simulink model "Linear_Moving_Setpoint_SS_PID"  (R2021b)
settings: Solver=VariableStepAuto  StartTime=tspan(1)  StopTime=tspan(2)  RelTol=1e-9
undefined symbols (not defined in the file): K1, K2, r_sim, x_0
settings Model: Creator=domin  LastModifiedBy=domin
settings SolverCC: AlgebraicLoopSolver=TrustRegion
settings DebuggingCC: SFMachineParentedDataDiag=warning

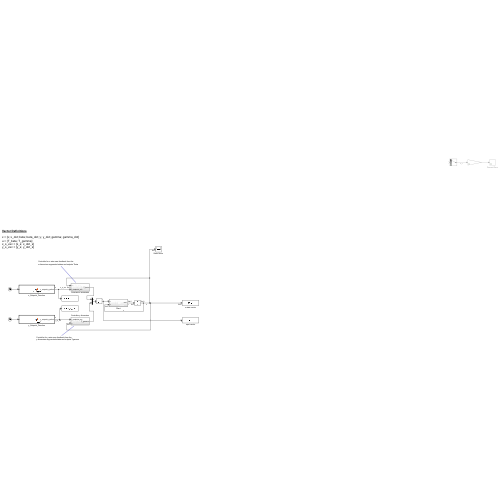
[thumbnail: Simulink's stored preview of the top-level diagram]
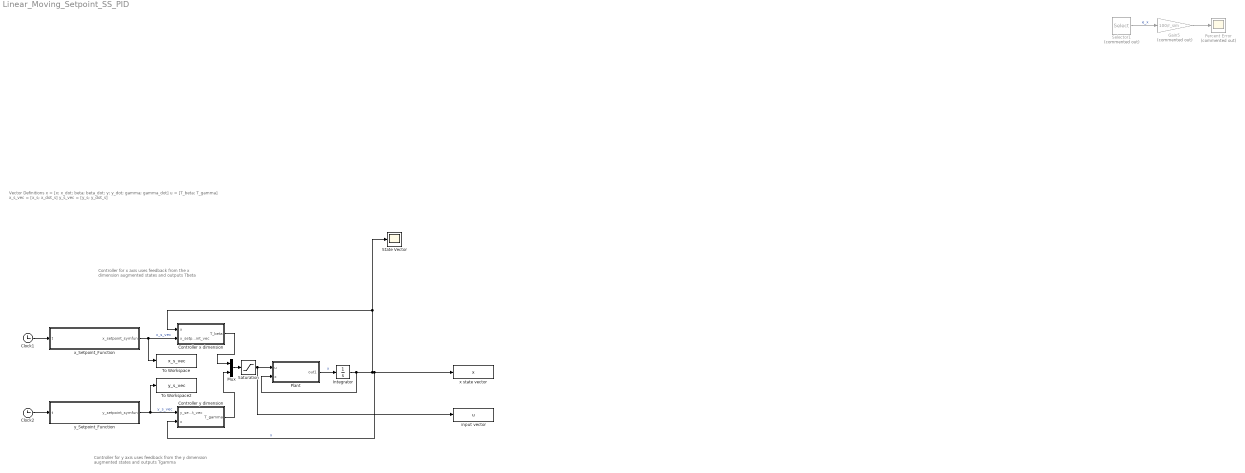
== system Linear_Moving_Setpoint_SS_PID ==
  note: Controller for y axis uses feedback from the
      | y dimension augmented states and outputs Tgamma
  note: Vector Definitions
      |
      | x = [x; x_dot; beta; beta_dot; y; y_dot; gamma; gamma_dot]
      | u = [T_beta; T_gamma]
      | x_s_vec = [x_s; x_dot_s]
      | y_s_vec = [y_s; y_dot_s]
  note: Controller for x axis uses feedback from the
      | x dimension augmented states and outputs Tbeta
  Clock1 : Clock
  Clock2 : Clock
  Controller x dimension : Subsystem
  Controller y dimension : Subsystem
  Gain5 : Gain  Commented=on  Gain=100/r_sim
  Integrator : Integrator  InitialCondition=x_0
  Mux : Mux  Inputs=2
  Percent Error : Scope  Commented=on
  Plant : Subsystem
  Saturation : Saturate  UpperLimit=73/1000  LowerLimit=-73/1000
  Selector1 : Selector  Commented=on  InputPortWidth=5  IndexOptions=Index vector (dialog)  Indices=[1]  OutputSizes=1
  State Vector : Scope
  To Workspace : ToWorkspace  VariableName=x_s_vec  SampleTime=-1
  To Workspace2 : ToWorkspace  VariableName=y_s_vec  SampleTime=-1
  input vector : ToWorkspace  VariableName=u  SampleTime=-1
  x state vector : ToWorkspace  VariableName=x  SampleTime=-1
  x_Setpoint_Function : MATLAB Function  TreatAsAtomicUnit=on
  y_Setpoint_Function : MATLAB Function  TreatAsAtomicUnit=on
  wires:
  x_Setpoint_Function/1(x_setpoint_symfun) -> To Workspace/1, Controller x dimension/2(x_setpoint_vec)  "x_s_vec"
  Integrator/1 -> Plant/2(x), Controller y dimension/2(x), x state vector/1, Controller x dimension/1(x), State Vector/1  "x"
  Plant/1(out1) -> Integrator/1  "x"
  Clock1/1 -> x_Setpoint_Function/1(t)
  Gain5/1 -> Percent Error/1
  Selector1/1 -> Gain5/1  "e_x"
  Clock2/1 -> y_Setpoint_Function/1(t)
  Mux/1 -> Saturation/1
  Controller x dimension/1(T_beta) -> Mux/1
  Controller y dimension/1(T_gamma) -> Mux/2
  y_Setpoint_Function/1(y_setpoint_symfun) -> To Workspace2/1, Controller y dimension/1(y_setpoint_vec)  "y_s_vec"
  Saturation/1 -> Plant/1(u), input vector/1

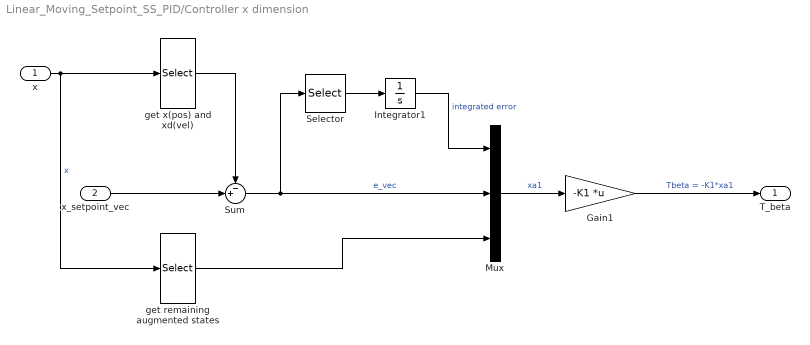
== system Linear_Moving_Setpoint_SS_PID/Controller x dimension ==
  x : Inport
  x_setpoint_vec : Inport  Port=2
  Gain1 : Gain  Gain=-K1  Multiplication=Matrix(K*u)
  Integrator1 : Integrator
  Mux : Mux  Inputs=3
  Selector : Selector  InputPortWidth=2  IndexOptions=Index vector (dialog)  Indices=[1 ]  OutputSizes=1
  Sum : Sum  Inputs=-+|
  get remaining augmented states : Selector  InputPortWidth=8  IndexOptions=Index vector (dialog)  Indices=[3,4]  OutputSizes=1
  get x(pos) and xd(vel) : Selector  InputPortWidth=8  IndexOptions=Index vector (dialog)  Indices=[1 2]  OutputSizes=1
  T_beta : Outport
  wires:
  get remaining augmented states/1 -> Mux/3
  Gain1/1 -> T_beta/1  "Tbeta = -K1*xa1"
  get x(pos) and xd(vel)/1 -> Sum/1
  Mux/1 -> Gain1/1  "xa1"
  Sum/1 -> Selector/1, Mux/2  "e_vec"
  x_setpoint_vec/1 -> Sum/2
  x/1 -> get x(pos) and xd(vel)/1, get remaining augmented states/1  "x"
  Selector/1 -> Integrator1/1
  Integrator1/1 -> Mux/1  "integrated error"

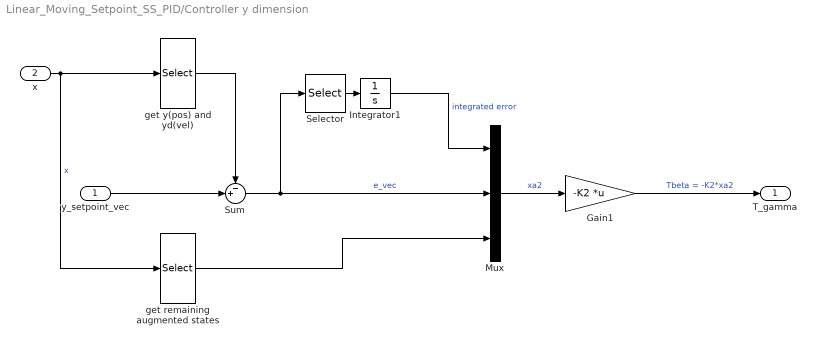
== system Linear_Moving_Setpoint_SS_PID/Controller y dimension ==
  y_setpoint_vec : Inport
  x : Inport  Port=2
  Gain1 : Gain  Gain=-K2  Multiplication=Matrix(K*u)
  Integrator1 : Integrator
  Mux : Mux  Inputs=3
  Selector : Selector  InputPortWidth=2  IndexOptions=Index vector (dialog)  Indices=[1 ]  OutputSizes=1
  Sum : Sum  Inputs=-+|
  get remaining augmented states : Selector  InputPortWidth=8  IndexOptions=Index vector (dialog)  Indices=[7,8]  OutputSizes=1
  get y(pos) and yd(vel) : Selector  InputPortWidth=8  IndexOptions=Index vector (dialog)  Indices=[5 6]  OutputSizes=1
  T_gamma : Outport
  wires:
  Integrator1/1 -> Mux/1  "integrated error"
  x/1 -> get y(pos) and yd(vel)/1, get remaining augmented states/1  "x"
  Gain1/1 -> T_gamma/1  "Tbeta = -K2*xa2"
  get y(pos) and yd(vel)/1 -> Sum/1
  Mux/1 -> Gain1/1  "xa2"
  get remaining augmented states/1 -> Mux/3
  Selector/1 -> Integrator1/1
  Sum/1 -> Selector/1, Mux/2  "e_vec"
  y_setpoint_vec/1 -> Sum/2

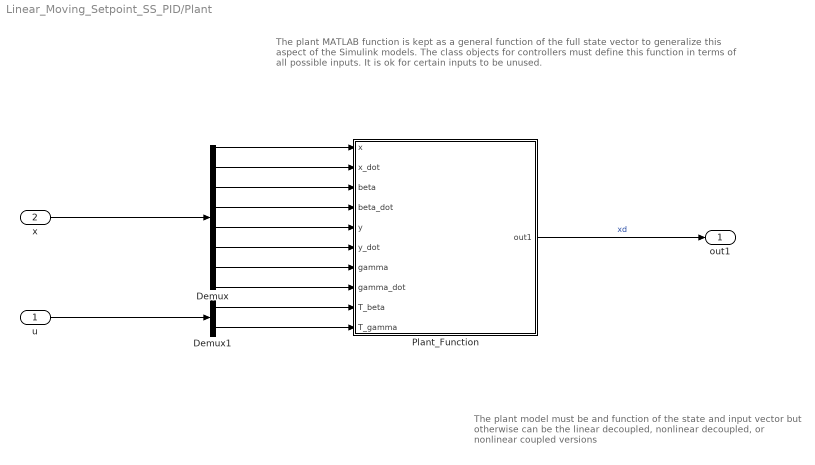
== system Linear_Moving_Setpoint_SS_PID/Plant ==
  note: The plant MATLAB function is kept as a general function of the full state vector
      | to generalize this aspect of the Simulink models. The class objects for controllers must define this function in terms of all possible inputs. It is ok for certain inputs to be unused.
  note: The plant model must be and function of the state and input vector
      |  but otherwise can be the linear decoupled, nonlinear decoupled,
      | or nonlinear coupled versions
  u : Inport
  x : Inport  Port=2
  Demux : Demux  Outputs=8
  Demux1 : Demux  Outputs=2
  Plant_Function : MATLAB Function  TreatAsAtomicUnit=on
  out1 : Outport
  wires:
  Demux1/1 -> Plant_Function/9(T_beta)
  Demux1/2 -> Plant_Function/10(T_gamma)
  Demux/5 -> Plant_Function/5(y)
  Demux/8 -> Plant_Function/8(gamma_dot)
  Demux/7 -> Plant_Function/7(gamma)
  Demux/1 -> Plant_Function/1(x)
  Demux/3 -> Plant_Function/3(beta)
  Demux/4 -> Plant_Function/4(beta_dot)
  Demux/2 -> Plant_Function/2(x_dot)
  Demux/6 -> Plant_Function/6(y_dot)
  x/1 -> Demux/1
  Plant_Function/1(out1) -> out1/1  "xd"
  u/1 -> Demux1/1

== matlab function Linear_Moving_Setpoint_SS_PID/Plant/Plant_Function ==
  data: x input; out1 output size=8; x_dot input; beta input; beta_dot input; y input; y_dot input; gamma input; gamma_dot input; T_beta input; T_gamma input
function out1 = xdot(x,x_dot,beta,beta_dot,y,y_dot,gamma,gamma_dot,T_beta,T_gamma)
%#codegen

%    This function was generated by the Symbolic Math Toolbox version 9.0.
%    08-Nov-2021 16:28:32

t2 = cos(beta);
t3 = cos(gamma);
t4 = sin(beta);
t5 = sin(gamma);
t6 = beta_dot.^2;
t7 = gamma_dot.^2;
t8 = x.^2;
t9 = x.^3;
t10 = y.^2;
t11 = y.^3;
t13 = y.^5;
t12 = t10.^2;
t14 = t3.^2;
t15 = t3.^3;
t17 = t3.^5;
t19 = t5.^2;
t20 = t5.^3;
t22 = t5.^5;
t29 = t3.*t5.*t8.*y.*6.615e-4;
t33 = t3.*t5.*y.*3.93855e-4;
t16 = t14.^2;
t18 = t14.^3;
t21 = t19.^2;
t24 = t3.*t11.*t20.*6.3e-3;
t25 = t5.*t11.*t15.*6.3e-3;
t27 = t8.*t19.*3.948e-3;
t28 = t12.*t14.*t19.*(6.3e+1./1.0e+3);
t31 = -t29;
t32 = t8.*t10.*t14.*t19.*(6.3e+1./1.0e+3);
t34 = t10.*t19.*3.93855e-3;
t35 = t8.*t14.*1.3784925e-2;
t37 = t3.*t8.*t20.*y.*6.9615e-3;
t38 = t5.*t8.*t15.*y.*6.9615e-3;
t39 = t3.*t20.*y.*1.53621e-4;
t40 = t5.*t15.*y.*1.53621e-4;
t44 = t14.*1.197923111e-3;
t45 = t8.*t14.*t19.*6.858495e-3;
t46 = t19.*6.079151925e-7;
t48 = t10.*t14.*t19.*2.070759405e-2;
t49 = t14.*t19.*4.674805062135e-4;
t23 = t12.*t21.*(6.3e+1./1.0e+3);
t26 = t8.*t10.*t21.*(6.3e+1./1.0e+3);
t30 = t8.*t21.*1.48176e-3;
t36 = t10.*t16.*1.916166e-2;
t41 = t8.*t16.*5.376735e-3;
t42 = t10.*t21.*1.54593405e-3;
t43 = t16.*4.672433922e-4;
t47 = t21.*2.371140135e-7;
t50 = t23+t24+t25+t26+t27+t28+t30+t31+t32+t33+t34+t35+t36+t37+t38+t39+t40+t41+t42+t43+t44+t45+t46+t47+t48+t49;
t51 = 1.0./t50;
et1 = T_beta.*t3.*(-2.123534875e-2)-T_beta.*t15.*8.28273225e-3+t4.*t14.*4.8049835404725e-3+t4.*t16.*1.8741576886695e-3+t4.*t19.*4.259748598875e-6+t4.*t21.*1.661491766025e-6-T_beta.*t3.*t19.*8.28273225e-3;
et2 = T_beta.*t10.*t15.*(-3.39675e-1)-T_beta.*t11.*t20.*(2.1e+1./4.0)+beta_dot.*gamma_dot.*t20.*5.4364987215e-8+beta_dot.*gamma_dot.*t22.*2.1204767493e-8-T_beta.*t5.*y.*3.282125e-1-T_beta.*t20.*y.*1.280175e-1-beta_dot.*t20.*y_dot.*1.04214033e-6-beta_dot.*t22.*y_dot.*4.06481166e-7;
et3 = t4.*t8.*t14.*9.659293875e-2+t4.*t8.*t16.*3.767555025e-2+t6.*t9.*t14.*9.846375e-3+t4.*t10.*t16.*7.685924085e-2+t4.*t8.*t19.*2.76642e-2+t6.*t9.*t16.*3.840525e-3+t4.*t8.*t21.*1.0382904e-2+t6.*t9.*t19.*2.82e-3+t4.*t10.*t21.*6.81378075e-5;
et4 = t6.*t9.*t21.*1.0584e-3+t4.*t14.*t19.*1.875819180435525e-3-t2.*t3.*x.*6.249563137125e-3-t2.*t15.*x.*2.437608101175e-3+t6.*t14.*x.*8.4655850125e-4+t7.*t14.*x.*3.854215798125e-5;
et5 = t6.*t16.*x.*3.6873769573125e-4+t7.*t16.*x.*1.503315903375e-5+t6.*t18.*x.*1.503315903375e-5+t6.*t19.*x.*4.342251375e-7+t6.*t21.*x.*1.693671525e-7-T_beta.*t5.*t11.*t14.*(2.1e+1./4.0)-T_beta.*t3.*t10.*t19.*3.39675e-1;
et6 = beta_dot.*gamma_dot.*t5.*t14.*(-3.66123403597875e-6)-beta_dot.*gamma_dot.*t5.*t16.*1.42804441695825e-6+beta_dot.*gamma_dot.*t8.*t20.*3.53064e-4-beta_dot.*gamma_dot.*t11.*t17.*2.708265e-2+beta_dot.*gamma_dot.*t8.*t22.*1.3251168e-4+beta_dot.*gamma_dot.*t10.*t20.*4.1354775e-5+beta_dot.*gamma_dot.*t10.*t22.*1.69998129e-5;
et7 = beta_dot.*gamma_dot.*t12.*t22.*6.615e-4-beta_dot.*gamma_dot.*t14.*t20.*1.40683964946525e-6+T_gamma.*t3.*t5.*x.*4.8525e-3-T_beta.*t5.*t14.*y.*1.280175e-1-beta_dot.*gamma_dot.*t15.*y.*1.6931170025e-3-beta_dot.*gamma_dot.*t17.*y.*6.603910755e-4-T_gamma.*t14.*x.*y.*3.39675e-1+T_gamma.*t19.*x.*y.*(3.0./4.0e+1);
et8 = beta_dot.*t5.*t14.*y_dot.*(-2.0471572661925e-3)-beta_dot.*t5.*t16.*y_dot.*7.984825542135e-4-beta_dot.*t8.*t20.*y_dot.*6.768e-3-beta_dot.*t8.*t22.*y_dot.*2.54016e-3-beta_dot.*t10.*t20.*y_dot.*3.93855e-3-beta_dot.*t10.*t22.*y_dot.*1.5528798e-3-beta_dot.*t12.*t22.*y_dot.*(6.3e+1./1.0e+3)-beta_dot.*t14.*t20.*y_dot.*7.988890353795e-4;
et9 = beta_dot.*t15.*x.*x_dot.*1.274120925e-3+beta_dot.*t17.*x.*x_dot.*4.96963935e-4-gamma_dot.*t3.*t5.*x_dot.*2.6756539425e-6-gamma_dot.*t5.*t15.*x_dot.*1.0436242635e-6-gamma_dot.*t3.*t20.*x_dot.*1.0436242635e-6-gamma_dot.*t11.*t21.*x_dot.*6.615e-4-gamma_dot.*t14.*x.*y_dot.*1.274120925e-3;
et10 = gamma_dot.*t16.*x.*y_dot.*(-4.96963935e-4)-gamma_dot.*t19.*x_dot.*y.*4.1354775e-5-gamma_dot.*t21.*x_dot.*y.*1.6130205e-5-t4.*t5.*t11.*t15.*8.71731315e-1-t3.*t4.*t11.*t20.*8.71731315e-1+t4.*t8.*t10.*t21.*4.4145e-1+t4.*t8.*t14.*t19.*4.805845425e-2+t6.*t9.*t10.*t21.*(9.0./2.0e+2);
et11 = t4.*t10.*t14.*t19.*7.69273786575e-2+t6.*t9.*t14.*t19.*4.898925e-3+t2.*t3.*t19.*x.*2.908211606325e-3+t2.*t3.*t21.*x.*1.679434722e-3-t6.*t10.*t14.*x.*3.057075e-5-t7.*t10.*t14.*x.*3.057075e-5+t6.*t10.*t16.*x.*1.37480415e-2-t2.*t11.*t20.*x.*1.545075;
et12 = t7.*t10.*t16.*x.*1.7614575e-4-t6.*t10.*t18.*x.*1.7614575e-4+t2.*t11.*t22.*x.*1.103625+t6.*t10.*t19.*x.*2.82e-3+t2.*t15.*t19.*x.*1.679434722e-3+t7.*t10.*t19.*x.*2.82e-3+t6.*t10.*t21.*x.*1.06534575e-3+t7.*t10.*t21.*x.*1.194525e-3+t6.*t12.*t21.*x.*(9.0./2.0e+2);
et13 = t6.*t14.*t19.*x.*3.322806719025e-4+t7.*t12.*t21.*x.*(9.0./2.0e+2)+t7.*t14.*t19.*x.*1.503315903375e-5+t6.*t14.*t21.*x.*7.1902404e-7+t6.*t16.*t19.*x.*1.575218307375e-5-t3.*t4.*t5.*y.*5.449773604275e-2;
et14 = t4.*t5.*t15.*y.*(-2.125654545105e-2)-t3.*t4.*t20.*y.*2.125654545105e-2-t2.*t5.*x.*y.*9.659293875e-2+t2.*t20.*x.*y.*4.494917475e-2+t2.*t22.*x.*y.*2.595726e-2+beta_dot.*gamma_dot.*t5.*t8.*t14.*1.23276615e-3+beta_dot.*gamma_dot.*t5.*t8.*t16.*4.8083373e-4;
et15 = beta_dot.*gamma_dot.*t5.*t10.*t14.*8.270955e-5-beta_dot.*gamma_dot.*t5.*t10.*t16.*2.6303717475e-5+beta_dot.*gamma_dot.*t5.*t12.*t16.*1.323e-3-beta_dot.*gamma_dot.*t3.*t11.*t21.*2.71626915e-2+beta_dot.*gamma_dot.*t8.*t10.*t22.*5.634e-3+beta_dot.*gamma_dot.*t8.*t14.*t20.*6.1334541e-4-beta_dot.*gamma_dot.*t10.*t14.*t20.*9.303904575e-6;
et16 = beta_dot.*gamma_dot.*t11.*t15.*t19.*(-5.42453415e-2)+beta_dot.*gamma_dot.*t12.*t14.*t20.*1.9845e-3-T_gamma.*t3.*t5.*t10.*x.*(2.1e+1./4.0)-beta_dot.*gamma_dot.*t3.*t19.*y.*1.698120930275e-3-beta_dot.*gamma_dot.*t8.*t15.*y.*1.969275e-2-beta_dot.*gamma_dot.*t3.*t21.*y.*6.62342830305e-4-beta_dot.*gamma_dot.*t8.*t17.*y.*7.68105e-3;
et17 = beta_dot.*gamma_dot.*t15.*t19.*y.*(-1.322733905805e-3)-beta_dot.*t5.*t8.*t14.*y_dot.*2.36313e-2-beta_dot.*t5.*t8.*t16.*y_dot.*9.21726e-3-beta_dot.*t5.*t10.*t16.*y_dot.*3.274578405e-2-beta_dot.*t3.*t11.*t21.*y_dot.*6.3e-3-beta_dot.*t8.*t10.*t22.*y_dot.*(2.7e+1./2.5e+2)-beta_dot.*t8.*t14.*t20.*y_dot.*1.175742e-2-beta_dot.*t10.*t14.*t20.*y_dot.*3.429866385e-2;
et18 = beta_dot.*t11.*t15.*t19.*y_dot.*(-6.3e-3)-beta_dot.*t12.*t14.*t20.*y_dot.*(6.3e+1./1.0e+3)+beta_dot.*t3.*t19.*x.*x_dot.*1.82454e-4+beta_dot.*t3.*t21.*x.*x_dot.*6.847848e-5+beta_dot.*t11.*t22.*x.*x_dot.*(9.0./2.0e+2)+beta_dot.*t15.*t19.*x.*x_dot.*5.65442415e-4-gamma_dot.*t5.*t10.*t15.*x_dot.*4.279905e-5-gamma_dot.*t3.*t10.*t20.*x_dot.*4.279905e-5-gamma_dot.*t11.*t14.*t19.*x_dot.*6.615e-4;
et19 = beta_dot.*t3.*t19.*y.*y_dot.*(-3.93855e-4)-beta_dot.*t3.*t21.*y.*y_dot.*1.53621e-4-beta_dot.*t15.*t19.*y.*y_dot.*1.53621e-4+beta_dot.*t20.*x.*x_dot.*y.*2.82e-3+beta_dot.*t22.*x.*x_dot.*y.*1.0584e-3-gamma_dot.*t10.*t21.*x.*y_dot.*4.5e-3-gamma_dot.*t14.*t19.*x.*y_dot.*4.96963935e-4-gamma_dot.*t14.*t19.*x_dot.*y.*1.6130205e-5+t4.*t8.*t10.*t14.*t19.*4.4145e-1;
et20 = t6.*t9.*t10.*t14.*t19.*(9.0./2.0e+2)-t3.*t5.*t6.*t11.*x.*4.725e-4-t3.*t5.*t7.*t11.*x.*4.725e-4-t2.*t3.*t10.*t19.*x.*1.076122665+t2.*t3.*t10.*t21.*x.*1.3817385e-1+t5.*t6.*t11.*t15.*x.*5.445e-3+t5.*t7.*t11.*t15.*x.*5.634e-3-t5.*t6.*t11.*t17.*x.*5.634e-3+t3.*t6.*t11.*t20.*x.*4.9725e-3+t3.*t7.*t11.*t20.*x.*5.634e-3+t3.*t6.*t11.*t22.*x.*4.9725e-3;
et21 = t2.*t10.*t15.*t19.*x.*1.3817385e-1+t2.*t11.*t14.*t20.*x.*1.103625+t6.*t10.*t14.*t19.*x.*3.165060525e-2+t7.*t10.*t14.*t19.*x.*1.37067075e-3+t6.*t10.*t14.*t21.*x.*7.109082e-3+t6.*t10.*t16.*t19.*x.*6.93293625e-3+t6.*t12.*t14.*t19.*x.*(9.0./2.0e+2)-t6.*t11.*t15.*t20.*x.*6.615e-4+t7.*t12.*t14.*t19.*x.*(9.0./2.0e+2)-t6.*t12.*t14.*t21.*x.*(9.0./2.0e+2);
et22 = t6.*t12.*t16.*t19.*x.*(-9.0./2.0e+2)-t3.*t4.*t5.*t8.*y.*4.635225e-3-t3.*t5.*t6.*t9.*y.*4.725e-4+t4.*t5.*t8.*t15.*y.*4.8780225e-2+t3.*t4.*t8.*t20.*y.*4.8780225e-2+t5.*t6.*t9.*t15.*y.*4.9725e-3+t3.*t6.*t9.*t20.*y.*4.9725e-3+t3.*t5.*t6.*x.*y.*1.41099225e-4+t3.*t5.*t7.*x.*y.*7.781596875e-4;
et23 = t2.*t5.*t14.*x.*y.*(-1.0083286366875e-1)+t2.*t5.*t16.*x.*y.*4.31997451875e-3+t5.*t6.*t15.*x.*y.*1.739399894625e-3+t5.*t7.*t15.*x.*y.*3.0963753e-4+t5.*t6.*t17.*x.*y.*6.71494035375e-4+t3.*t6.*t20.*x.*y.*8.1958275e-5+t3.*t7.*t20.*x.*y.*3.0963753e-4;
et24 = t3.*t6.*t22.*x.*y.*1.11132e-5+t2.*t14.*t20.*x.*y.*3.027723451875e-2+t6.*t15.*t20.*x.*y.*6.82607235375e-4-beta_dot.*t8.*t10.*t14.*t20.*y_dot.*(2.7e+1./2.5e+2)-beta_dot.*t3.*t10.*t19.*x.*x_dot.*4.725e-4+beta_dot.*t3.*t10.*t21.*x.*x_dot.*1.0134e-2+beta_dot.*t10.*t15.*t19.*x.*x_dot.*1.0134e-2+beta_dot.*t11.*t14.*t20.*x.*x_dot.*(9.0./2.0e+2)+beta_dot.*t3.*t8.*t19.*y.*y_dot.*1.134e-3-beta_dot.*t3.*t8.*t21.*y.*y_dot.*1.1934e-2;
et25 = beta_dot.*t8.*t15.*t19.*y.*y_dot.*(-1.1934e-2)+beta_dot.*t5.*t14.*x.*x_dot.*y.*1.966217925e-2+beta_dot.*t5.*t16.*x.*x_dot.*y.*8.14834575e-3+beta_dot.*t14.*t20.*x.*x_dot.*y.*9.20674575e-3-gamma_dot.*t10.*t14.*t19.*x.*y_dot.*4.5e-3-gamma_dot.*t3.*t5.*x.*y.*y_dot.*1.969275e-2-gamma_dot.*t5.*t15.*x.*y.*y_dot.*7.9722e-3-gamma_dot.*t3.*t20.*x.*y.*y_dot.*7.9722e-3+beta_dot.*gamma_dot.*t5.*t8.*t10.*t14.*9.45e-4;
et26 = beta_dot.*gamma_dot.*t5.*t8.*t10.*t16.*(-9.945e-3)-beta_dot.*gamma_dot.*t3.*t8.*t11.*t21.*(9.0./1.0e+2)-beta_dot.*gamma_dot.*t8.*t10.*t14.*t20.*4.311e-3-beta_dot.*gamma_dot.*t8.*t11.*t15.*t19.*(9.0./1.0e+2)-beta_dot.*gamma_dot.*t3.*t8.*t19.*y.*5.699157e-3-beta_dot.*gamma_dot.*t3.*t8.*t21.*y.*1.494243e-3-beta_dot.*gamma_dot.*t8.*t15.*t19.*y.*9.175293e-3;
et27 = T_beta.*(-4.594975e-1)-T_beta.*t14.*1.792245e-1-T_beta.*t19.*1.792245e-1-t3.*t4.*7.7660722755e-2-t4.*t15.*3.0291142401e-2-t2.*x.*1.3523011425e-1-T_beta.*t10.*t14.*(1.47e+2./2.0e+1)-T_beta.*t10.*t19.*(1.47e+2./2.0e+1)+T_gamma.*t5.*x.*(2.1e+1./2.0e+2)-gamma_dot.*t5.*x_dot.*5.7896685e-5;
et28 = gamma_dot.*t20.*x_dot.*(-2.2582287e-5)-t3.*t4.*t19.*3.0291142401e-2-t4.*t10.*t15.*1.2422403-t4.*t11.*t20.*6.1803e-1-t3.*t6.*x.*1.969275e-4+t3.*t7.*x.*8.339879625e-4-t2.*t14.*x.*5.274577035e-2+t2.*t19.*x.*6.292884465e-2;
et29 = t6.*t15.*x.*7.571774625e-4+t7.*t15.*x.*3.252924675e-4+t2.*t21.*x.*3.6340164e-2+t6.*t17.*x.*3.252924675e-4-t4.*t5.*y.*3.86371755e-2-t4.*t20.*y.*1.50702201e-2-beta_dot.*gamma_dot.*t3.*t5.*2.3973060455575e-3;
et30 = beta_dot.*gamma_dot.*t5.*t15.*(-9.350561806365e-4)-beta_dot.*gamma_dot.*t3.*t20.*9.350561806365e-4+beta_dot.*gamma_dot.*t11.*t16.*6.3e-3-beta_dot.*gamma_dot.*t11.*t21.*6.9615e-3+beta_dot.*gamma_dot.*t14.*y.*3.93855e-4+beta_dot.*gamma_dot.*t16.*y.*1.53621e-4-beta_dot.*gamma_dot.*t19.*y.*4.35209775e-4-beta_dot.*gamma_dot.*t21.*y.*1.69751205e-4;
et31 = T_gamma.*t3.*x.*y.*(-1.47e+2./2.0e+1)+beta_dot.*t3.*t5.*y_dot.*1.39030815e-4+beta_dot.*t5.*t15.*y_dot.*5.4228213e-5+beta_dot.*t3.*t20.*y_dot.*5.4228213e-5+beta_dot.*t11.*t21.*y_dot.*(6.3e+1./1.0e+3)+beta_dot.*t14.*x.*x_dot.*2.756985e-2+beta_dot.*t16.*x.*x_dot.*1.075347e-2+beta_dot.*t19.*x.*x_dot.*3.948e-3+beta_dot.*t21.*x.*x_dot.*1.48176e-3;
et32 = gamma_dot.*t5.*t14.*x_dot.*(-2.2582287e-5)-gamma_dot.*t10.*t20.*x_dot.*9.261e-4+beta_dot.*t19.*y.*y_dot.*3.93855e-3+beta_dot.*t21.*y.*y_dot.*1.53621e-3-gamma_dot.*t3.*x.*y_dot.*2.756985e-2-gamma_dot.*t15.*x.*y_dot.*1.075347e-2-t4.*t5.*t11.*t14.*6.1803e-1-t3.*t4.*t10.*t19.*1.2422403-t3.*t6.*t10.*x.*6.615e-4;
et33 = t3.*t7.*t10.*x.*(-6.615e-4)-t3.*t6.*t19.*x.*3.53565e-5+t3.*t7.*t19.*x.*3.252924675e-4+t3.*t6.*t21.*x.*1.555848e-5-t2.*t10.*t19.*x.*2.163105+t6.*t10.*t15.*x.*1.323e-3+t7.*t10.*t15.*x.*3.8115e-3+t2.*t10.*t21.*x.*1.545075-t6.*t10.*t17.*x.*3.8115e-3;
et34 = t2.*t14.*t19.*x.*3.6340164e-2+t7.*t11.*t20.*x.*(6.3e+1./1.0e+3)+t6.*t15.*t19.*x.*3.408509475e-4-t4.*t5.*t14.*y.*1.50702201e-2+t5.*t6.*x.*y.*9.45e-6+t5.*t7.*x.*y.*3.948e-3-t6.*t20.*x.*y.*5.445e-5+t7.*t20.*x.*y.*1.672335e-3+beta_dot.*gamma_dot.*t3.*t5.*t10.*7.8771e-3;
et35 = beta_dot.*gamma_dot.*t5.*t10.*t15.*(-3.527425095e-2)+beta_dot.*gamma_dot.*t5.*t12.*t15.*(6.3e+1./5.0e+2)-beta_dot.*gamma_dot.*t3.*t10.*t20.*3.527425095e-2+beta_dot.*gamma_dot.*t3.*t12.*t20.*(6.3e+1./5.0e+2)-beta_dot.*gamma_dot.*t11.*t14.*t19.*6.615e-4-beta_dot.*gamma_dot.*t14.*t19.*y.*1.6130205e-5+beta_dot.*t5.*t10.*t15.*y_dot.*2.2239e-3+beta_dot.*t3.*t10.*t20.*y_dot.*2.2239e-3+beta_dot.*t11.*t14.*t19.*y_dot.*(6.3e+1./1.0e+3)+beta_dot.*t10.*t21.*x.*x_dot.*(6.3e+1./1.0e+3);
et36 = beta_dot.*t14.*t19.*x.*x_dot.*1.223523e-2-gamma_dot.*t5.*t10.*t14.*x_dot.*9.261e-4+beta_dot.*t14.*t19.*y.*y_dot.*1.53621e-3-gamma_dot.*t3.*t19.*x.*y_dot.*1.075347e-2-gamma_dot.*t20.*x.*y.*y_dot.*6.3e-3+t5.*t7.*t11.*t14.*x.*(6.3e+1./1.0e+3)+t3.*t6.*t10.*t19.*x.*6.615e-4-t5.*t6.*t11.*t16.*x.*(6.3e+1./1.0e+3)+t3.*t7.*t10.*t19.*x.*3.8115e-3+t3.*t6.*t10.*t21.*x.*6.9615e-3;
et37 = t2.*t10.*t14.*t19.*x.*1.545075+t6.*t10.*t15.*t19.*x.*3.15e-3-t6.*t11.*t14.*t20.*x.*(6.3e+1./1.0e+3)-t2.*t3.*t5.*x.*y.*1.3666188375+t2.*t5.*t15.*x.*y.*9.34770375e-2+t2.*t3.*t20.*x.*y.*9.34770375e-2+t5.*t6.*t14.*x.*y.*2.356045425e-2+t5.*t7.*t14.*x.*y.*1.672335e-3+t5.*t6.*t16.*x.*y.*9.50230575e-3;
et38 = t6.*t14.*t20.*x.*y.*9.50230575e-3+beta_dot.*t10.*t14.*t19.*x.*x_dot.*(6.3e+1./1.0e+3)-beta_dot.*t3.*t5.*x.*x_dot.*y.*6.615e-4+beta_dot.*t5.*t15.*x.*x_dot.*y.*1.01115e-2+beta_dot.*t3.*t20.*x.*x_dot.*y.*1.01115e-2-gamma_dot.*t5.*t14.*x.*y.*y_dot.*6.3e-3;
et39 = T_gamma.*t14.*2.9518081e-2+T_gamma.*t19.*1.49796675e-5-t2.*t20.*1.537489879183125e-6-t2.*t22.*1.852002642301875e-6+T_gamma.*t8.*t14.*3.39675e-1+T_gamma.*t8.*t19.*2.205e-2+T_gamma.*t10.*t19.*9.705e-2+T_beta.*t5.*x.*3.29231525e-1;
et40 = T_beta.*t20.*x.*1.22145975e-1+beta_dot.*t20.*x_dot.*1.043488500075e-6+beta_dot.*t22.*x_dot.*3.98713138425e-7+t2.*t5.*t8.*9.68928378075e-2-t2.*t5.*t14.*3.02969013099975e-3-t2.*t5.*t16.*3.64945109814225e-3;
et41 = t5.*t6.*t15.*(-3.565874746455e-6)-t5.*t6.*t17.*1.562456127645e-6-t3.*t6.*t20.*1.8095897917125e-9-t2.*t8.*t20.*5.69186574075e-2-t3.*t6.*t22.*7.929063300375e-10;
et42 = t2.*t8.*t22.*(-3.6340164e-2)-t2.*t10.*t20.*9.9610617375e-3+t6.*t11.*t16.*1.36869e-2-t2.*t10.*t22.*1.206685917e-2+t7.*t11.*t16.*1.36869e-2-t6.*t11.*t18.*1.36869e-2-t2.*t12.*t22.*4.4145e-1-t2.*t14.*t20.*3.651303100784552e-3;
et43 = t6.*t11.*t19.*2.8219845e-3+t7.*t11.*t19.*2.8219845e-3+t6.*t11.*t21.*1.05391125e-3+t7.*t11.*t21.*1.230057e-3+t6.*t13.*t21.*(9.0./2.0e+2)-t6.*t15.*t20.*1.563249033975038e-6+t7.*t13.*t21.*(9.0./2.0e+2)-t2.*t15.*y.*8.6871712383e-3;
et44 = t6.*t14.*y.*8.5831599229e-4+t7.*t14.*y.*8.5831599229e-4-t6.*t16.*y.*5.3987794558e-4+t7.*t16.*y.*3.72013363725e-4-t6.*t18.*y.*2.64862729695e-4+t6.*t19.*y.*4.35573307575e-7;
et45 = t7.*t19.*y.*4.35573307575e-7+t6.*t21.*y.*1.61599124925e-7+t7.*t21.*y.*1.887872214375e-7+T_beta.*t5.*t14.*x.*1.22145975e-1+T_beta.*t10.*t20.*x.*(2.1e+1./4.0)+T_gamma.*t3.*t5.*y.*9.705e-3+T_beta.*t15.*x.*y.*3.39675e-1+beta_dot.*t5.*t14.*x_dot.*2.05623910329e-3;
et46 = beta_dot.*t5.*t16.*x_dot.*7.8568143891e-4+beta_dot.*t8.*t20.*x_dot.*3.948e-3+beta_dot.*t8.*t22.*x_dot.*1.48176e-3+beta_dot.*t10.*t20.*x_dot.*6.7605345e-3+beta_dot.*t10.*t22.*x_dot.*2.5998453e-3+beta_dot.*t12.*t22.*x_dot.*(2.7e+1./2.5e+2)+beta_dot.*t14.*t20.*x_dot.*7.86080152048425e-4+beta_dot.*t17.*x_dot.*y.*1.77108486e-3;
et47 = gamma_dot.*t11.*t21.*y_dot.*(-5.823e-3)+gamma_dot.*t19.*x.*x_dot.*4.148317215e-5+gamma_dot.*t21.*x.*x_dot.*1.539039285e-5-gamma_dot.*t16.*y.*y_dot.*1.77108486e-3-gamma_dot.*t21.*y.*y_dot.*8.9878005e-7+t3.*t5.*t6.*t8.*1.41099225e-4-t3.*t5.*t7.*t8.*5.97555217875e-4;
et48 = t3.*t5.*t6.*t10.*2.8219845e-4+t3.*t5.*t7.*t10.*2.8219845e-4+t2.*t5.*t8.*t14.*1.08384436125e-3-t2.*t5.*t8.*t16.*4.199552476875e-2-t2.*t5.*t10.*t14.*2.8561815e-3-t2.*t5.*t10.*t16.*1.34268489e-1-t5.*t6.*t8.*t15.*5.86240725e-4;
et49 = t2.*t3.*t11.*t19.*(-2.8561815e-2)-t5.*t7.*t8.*t15.*2.21694944625e-4-t5.*t6.*t8.*t17.*2.3967468e-4-t5.*t6.*t10.*t15.*1.775019e-4-t2.*t3.*t11.*t21.*4.4145e-2+t3.*t6.*t8.*t20.*1.0894275e-5+t5.*t7.*t10.*t15.*1.22311125e-4-t3.*t7.*t8.*t20.*2.21694944625e-4;
et50 = t5.*t6.*t10.*t17.*1.626517905e-3+t5.*t6.*t12.*t15.*4.5e-3-t3.*t6.*t8.*t22.*1.555848e-5+t3.*t6.*t10.*t20.*9.297261225e-5+t5.*t7.*t12.*t15.*4.5e-3+t2.*t8.*t10.*t20.*1.545075+t3.*t7.*t10.*t20.*1.22311125e-4-t5.*t6.*t12.*t17.*4.5e-3-t3.*t6.*t10.*t22.*4.26745935e-6+t3.*t6.*t12.*t20.*4.5e-3;
et51 = t2.*t8.*t10.*t22.*(-1.545075)+t3.*t7.*t12.*t20.*4.5e-3+t3.*t6.*t12.*t22.*5.634e-3-t2.*t8.*t14.*t20.*7.833568876875e-2-t2.*t10.*t14.*t20.*1.4633534817e-1+t6.*t8.*t11.*t21.*(9.0./2.0e+2)-t2.*t11.*t15.*t19.*4.4145e-2-t2.*t12.*t14.*t20.*4.4145e-1-t6.*t8.*t15.*t20.*2.5523316e-4+t6.*t11.*t14.*t19.*1.191882675e-2;
et52 = t6.*t10.*t15.*t20.*1.62225044565e-3+t7.*t11.*t14.*t19.*1.4916957e-2-t6.*t11.*t14.*t21.*3.143655e-4-t6.*t11.*t16.*t19.*1.40012655e-2+t6.*t13.*t14.*t19.*(9.0./2.0e+2)+t6.*t12.*t15.*t20.*1.134e-3+t7.*t13.*t14.*t19.*(9.0./2.0e+2)-t6.*t13.*t14.*t21.*(9.0./2.0e+2)-t6.*t13.*t16.*t19.*(9.0./2.0e+2)+t3.*t4.*t5.*x.*5.564417256945e-2;
et53 = t4.*t5.*t15.*x.*2.064417042555e-2+t3.*t4.*t20.*x.*2.064417042555e-2+t4.*t11.*t21.*x.*4.4145e-1-t2.*t3.*t19.*y.*1.00051468989525e-3-t2.*t3.*t21.*y.*1.19987213625e-3+t6.*t8.*t14.*y.*9.87694575e-3+t7.*t8.*t14.*y.*9.87694575e-3;
et54 = t6.*t8.*t16.*y.*(-6.0669915e-3)+t7.*t8.*t16.*y.*3.66437925e-3-t6.*t8.*t18.*y.*3.66437925e-3+t6.*t8.*t19.*y.*2.8219845e-3+t6.*t8.*t21.*y.*1.0469655e-3-t2.*t15.*t19.*y.*1.19987213625e-3+t7.*t8.*t21.*y.*4.002075e-5;
et55 = t6.*t14.*t19.*y.*3.1699167875235e-4+t7.*t14.*t19.*y.*3.722021509464375e-4-t6.*t14.*t21.*y.*6.481177534125e-7-t6.*t16.*t19.*y.*2.655108474484125e-4+t4.*t16.*x.*y.*5.740924815e-2;
et56 = t4.*t19.*x.*y.*2.7683667945e-2+t4.*t21.*x.*y.*1.0270731555e-2+T_beta.*t5.*t10.*t14.*x.*(2.1e+1./4.0)+T_gamma.*t3.*t5.*t8.*y.*(2.1e+1./4.0)+beta_dot.*gamma_dot.*t3.*t19.*x.*1.717677953134925e-3+beta_dot.*gamma_dot.*t3.*t21.*x.*6.37264151182575e-4-beta_dot.*gamma_dot.*t10.*t17.*x.*2.9115e-4+beta_dot.*gamma_dot.*t11.*t22.*x.*4.9725e-3;
et57 = beta_dot.*gamma_dot.*t15.*t19.*x.*6.37264151182575e-4+T_beta.*t3.*t19.*x.*y.*3.39675e-1+beta_dot.*gamma_dot.*t20.*x.*y.*3.1182928725e-4+beta_dot.*gamma_dot.*t22.*x.*y.*1.1568968775e-4+beta_dot.*t5.*t8.*t14.*x_dot.*3.90797925e-3+beta_dot.*t5.*t8.*t16.*x_dot.*1.71235575e-3+beta_dot.*t5.*t10.*t16.*x_dot.*3.343086e-2;
et58 = beta_dot.*t3.*t11.*t21.*x_dot.*1.6623e-2+beta_dot.*t8.*t10.*t22.*x_dot.*(6.3e+1./1.0e+3)+beta_dot.*t8.*t14.*t20.*x_dot.*3.19411575e-3+beta_dot.*t10.*t14.*t20.*x_dot.*3.60307053e-2+beta_dot.*t11.*t15.*t19.*x_dot.*1.6623e-2+beta_dot.*t12.*t14.*t20.*x_dot.*(2.7e+1./2.5e+2)-beta_dot.*t3.*t19.*x.*y_dot.*9.961605285e-5+beta_dot.*t3.*t19.*x_dot.*y.*6.7605345e-4;
et59 = beta_dot.*t3.*t21.*x.*y_dot.*(-3.695788215e-5)+beta_dot.*t3.*t21.*x_dot.*y.*2.5921633005e-4-beta_dot.*t11.*t22.*x.*y_dot.*(9.0./2.0e+2)-beta_dot.*t15.*t19.*x.*y_dot.*3.695788215e-5+beta_dot.*t15.*t19.*x_dot.*y.*2.03030119005e-3+gamma_dot.*t3.*t5.*t8.*y_dot.*1.97538915e-2+gamma_dot.*t5.*t8.*t15.*y_dot.*7.3287585e-3;
et60 = gamma_dot.*t5.*t10.*t15.*y_dot.*(-5.823e-4)+gamma_dot.*t3.*t8.*t20.*y_dot.*7.3287585e-3-gamma_dot.*t3.*t10.*t20.*y_dot.*5.823e-4-gamma_dot.*t11.*t14.*t19.*y_dot.*5.823e-3+gamma_dot.*t10.*t21.*x.*x_dot.*6.615e-4+gamma_dot.*t14.*t19.*x.*x_dot.*1.539039285e-5-beta_dot.*t20.*x.*y.*y_dot.*2.8219845e-3-beta_dot.*t22.*x.*y.*y_dot.*1.0469655e-3;
et61 = gamma_dot.*t8.*t21.*y.*y_dot.*(-1.323e-3)-gamma_dot.*t14.*t19.*y.*y_dot.*1.77198364005e-3+t5.*t6.*t8.*t10.*t15.*4.5e-3-t5.*t7.*t8.*t10.*t15.*6.615e-4+t5.*t6.*t8.*t10.*t17.*6.615e-4+t3.*t6.*t8.*t10.*t20.*4.5e-3-t3.*t7.*t8.*t10.*t20.*6.615e-4+t3.*t6.*t8.*t10.*t22.*6.615e-4-t2.*t8.*t10.*t14.*t20.*1.545075+t6.*t8.*t11.*t14.*t19.*(9.0./2.0e+2)+t6.*t8.*t10.*t15.*t20.*1.323e-3;
et62 = t4.*t5.*t10.*t15.*x.*9.15876315e-1+t3.*t4.*t10.*t20.*x.*9.15876315e-1+t4.*t11.*t14.*t19.*x.*4.4145e-1+t2.*t3.*t8.*t19.*y.*1.052196075-t2.*t3.*t8.*t21.*y.*1.86954075e-1-t2.*t8.*t15.*t19.*y.*1.86954075e-1-t6.*t8.*t14.*t19.*y.*1.4890026e-2+t7.*t8.*t14.*t19.*y.*3.7044e-3;
et63 = t6.*t8.*t14.*t21.*y.*(-7.36877925e-3)-t6.*t8.*t16.*t19.*y.*1.10331585e-2+t4.*t14.*t19.*x.*y.*6.7679979705e-2-beta_dot.*gamma_dot.*t5.*t14.*x.*y.*2.8219845e-4+beta_dot.*gamma_dot.*t5.*t16.*x.*y.*1.667467457475e-3+beta_dot.*gamma_dot.*t14.*t20.*x.*y.*1.783157145225e-3+beta_dot.*t8.*t10.*t14.*t20.*x_dot.*(6.3e+1./1.0e+3);
et64 = beta_dot.*t3.*t8.*t19.*x_dot.*y.*(-6.615e-4)+beta_dot.*t3.*t8.*t21.*x_dot.*y.*7.623e-3-beta_dot.*t3.*t10.*t21.*x.*y_dot.*4.5e-3+beta_dot.*t8.*t15.*t19.*x_dot.*y.*7.623e-3-beta_dot.*t10.*t15.*t19.*x.*y_dot.*4.5e-3-beta_dot.*t11.*t14.*t20.*x.*y_dot.*(9.0./2.0e+2)+gamma_dot.*t10.*t14.*t19.*x.*x_dot.*6.615e-4-beta_dot.*t5.*t16.*x.*y.*y_dot.*1.0277595e-4-beta_dot.*t14.*t20.*x.*y.*y_dot.*1.14974145e-3-gamma_dot.*t8.*t14.*t19.*y.*y_dot.*1.323e-3;
et65 = gamma_dot.*t5.*t15.*x.*x_dot.*y.*4.279905e-5+gamma_dot.*t3.*t20.*x.*x_dot.*y.*4.279905e-5-beta_dot.*gamma_dot.*t3.*t10.*t19.*x.*5.643969e-3-beta_dot.*gamma_dot.*t5.*t11.*t16.*x.*1.0323e-2+beta_dot.*gamma_dot.*t3.*t10.*t21.*x.*2.5618269e-2-beta_dot.*gamma_dot.*t3.*t12.*t21.*x.*(9.0./1.0e+2)+beta_dot.*gamma_dot.*t10.*t15.*t19.*x.*2.5327119e-2-beta_dot.*gamma_dot.*t11.*t14.*t20.*x.*5.3505e-3-beta_dot.*gamma_dot.*t12.*t15.*t19.*x.*(9.0./1.0e+2);
et66 = T_gamma.*t14.*6.38722e-1+T_gamma.*t19.*3.24135e-4+t2.*t20.*5.890513458375e-5-t2.*t22.*4.12233735375e-6+T_gamma.*t8.*t14.*(1.47e+2./2.0e+1)+T_gamma.*t8.*t19.*(2.1e+1./1.0e+1)+T_gamma.*t10.*t19.*(2.1e+1./1.0e+1)+T_beta.*t5.*x.*2.205e-2-T_beta.*t20.*x.*1.2705e-1+beta_dot.*t20.*x_dot.*2.917215e-8;
et67 = beta_dot.*t22.*x_dot.*(-1.6808715e-7)+t2.*t5.*t8.*6.489315e-3+t2.*t5.*t14.*1.160751087405e-1-t2.*t5.*t16.*8.1232435845e-3-t5.*t6.*t15.*1.19731951871e-3-t5.*t6.*t17.*4.7072123349e-4;
et68 = t3.*t6.*t20.*(-6.07608884925e-7)+t2.*t8.*t20.*3.39607485e-1-t3.*t6.*t22.*2.38878928575e-7+t2.*t10.*t20.*3.81633525e-1-t2.*t10.*t22.*2.6707725e-2-t2.*t14.*t20.*8.12736592185375e-3+t6.*t11.*t19.*1.89e-4+t7.*t11.*t19.*1.89e-4;
et69 = t6.*t11.*t21.*(-1.089e-3)+t7.*t11.*t21.*2.7225e-3-t6.*t15.*t20.*4.70960112418575e-4-t2.*t15.*y.*1.879758846e-1+t6.*t14.*y.*5.748498e-5+t7.*t14.*y.*5.748498e-5-t6.*t16.*y.*3.8870796e-4+t7.*t16.*y.*8.2805745e-4;
et70 = t6.*t18.*y.*1.49050341e-3+t6.*t19.*y.*2.917215e-8+t7.*t19.*y.*2.917215e-8-t6.*t21.*y.*1.6808715e-7+t7.*t21.*y.*4.20217875e-7-T_beta.*t5.*t14.*x.*1.2705e-1+T_gamma.*t3.*t5.*y.*(2.1e+1./1.0e+2)+T_beta.*t15.*x.*y.*(1.47e+2./2.0e+1)+beta_dot.*t5.*t14.*x_dot.*5.748498e-5;
et71 = beta_dot.*t5.*t16.*x_dot.*(-3.3122298e-4)+beta_dot.*t10.*t20.*x_dot.*1.89e-4-beta_dot.*t10.*t22.*x_dot.*1.089e-3-beta_dot.*t14.*t20.*x_dot.*3.3139106715e-4+beta_dot.*t17.*x_dot.*y.*3.832332e-2-gamma_dot.*t11.*t21.*y_dot.*(6.3e+1./5.0e+2)+gamma_dot.*t19.*x.*x_dot.*2.7783e-6-gamma_dot.*t21.*x.*x_dot.*1.60083e-5-gamma_dot.*t16.*y.*y_dot.*3.832332e-2;
et72 = gamma_dot.*t21.*y.*y_dot.*(-1.94481e-5)+t3.*t5.*t6.*t8.*9.45e-6-t3.*t5.*t7.*t8.*4.002075e-5+t3.*t5.*t6.*t10.*1.89e-5+t3.*t5.*t7.*t10.*1.89e-5+t2.*t5.*t8.*t14.*1.2983265225-t2.*t5.*t8.*t16.*9.34770375e-2-t2.*t5.*t10.*t14.*6.1803e-2-t5.*t6.*t8.*t15.*1.387245e-2;
et73 = t2.*t3.*t11.*t19.*(-6.1803e-1)+t5.*t7.*t8.*t15.*2.3059575e-4-t5.*t6.*t8.*t17.*5.18616e-3-t5.*t6.*t10.*t15.*1.278e-4-t3.*t6.*t8.*t20.*4.00245e-3+t5.*t7.*t10.*t15.*2.7225e-4+t3.*t7.*t8.*t20.*2.3059575e-4+t5.*t6.*t10.*t17.*1.965171e-2-t3.*t6.*t8.*t22.*1.48176e-3;
et74 = t3.*t6.*t10.*t20.*(-4.0454655e-3)+t3.*t7.*t10.*t20.*2.7225e-4-t3.*t6.*t10.*t22.*1.53792045e-3+t3.*t6.*t12.*t22.*(6.3e+1./1.0e+3)-t2.*t8.*t14.*t20.*9.34770375e-2-t2.*t10.*t14.*t20.*2.6707725e-2-t6.*t8.*t15.*t20.*6.66792e-3-t6.*t11.*t14.*t19.*1.278e-3+t6.*t10.*t15.*t20.*1.811378955e-2;
et75 = t7.*t11.*t14.*t19.*2.7225e-3+t6.*t11.*t14.*t21.*1.12005e-2+t6.*t11.*t16.*t19.*1.12005e-2+t6.*t12.*t15.*t20.*(6.3e+1./1.0e+3)+t3.*t4.*t5.*x.*3.7267209e-3-t4.*t5.*t15.*x.*2.14730109e-2-t3.*t4.*t20.*x.*2.14730109e-2+t2.*t3.*t19.*y.*3.80679595695e-2-t2.*t3.*t21.*y.*2.6707725e-3;
et76 = t6.*t8.*t14.*y.*6.615e-4+t7.*t8.*t14.*y.*6.615e-4-t6.*t8.*t16.*y.*1.323e-3-t7.*t8.*t16.*y.*3.8115e-3+t6.*t8.*t18.*y.*3.8115e-3+t6.*t8.*t19.*y.*1.89e-4-t6.*t8.*t21.*y.*1.089e-3-t2.*t15.*t19.*y.*2.6707725e-3+t7.*t8.*t21.*y.*3.8115e-3-t6.*t14.*t19.*y.*7.250767893e-4;
et77 = t7.*t14.*t19.*y.*8.28477667875e-4-t6.*t14.*t21.*y.*1.54008057825e-4+t6.*t16.*t19.*y.*1.336495352175e-3+t4.*t16.*x.*y.*1.2422403+t4.*t19.*x.*y.*1.85409e-3-t4.*t21.*x.*y.*1.068309e-2+beta_dot.*gamma_dot.*t3.*t19.*x.*1.1504001285e-4;
et78 = beta_dot.*gamma_dot.*t3.*t21.*x.*(-6.6284959785e-4)-beta_dot.*gamma_dot.*t10.*t17.*x.*6.3e-3-beta_dot.*gamma_dot.*t15.*t19.*x.*6.6284959785e-4+T_beta.*t3.*t19.*x.*y.*(1.47e+2./2.0e+1)+beta_dot.*gamma_dot.*t20.*x.*y.*2.08845e-5-beta_dot.*gamma_dot.*t22.*x.*y.*1.203345e-4-beta_dot.*t5.*t8.*t14.*x_dot.*6.615e-4+beta_dot.*t5.*t8.*t16.*x_dot.*3.8115e-3+beta_dot.*t5.*t10.*t16.*x_dot.*1.26e-2;
et79 = beta_dot.*t3.*t11.*t21.*x_dot.*(6.3e+1./5.0e+2)+beta_dot.*t8.*t14.*t20.*x_dot.*3.8115e-3+beta_dot.*t10.*t14.*t20.*x_dot.*1.1511e-2+beta_dot.*t11.*t15.*t19.*x_dot.*(6.3e+1./5.0e+2)-beta_dot.*t3.*t19.*x.*y_dot.*6.6717e-6+beta_dot.*t3.*t19.*x_dot.*y.*1.89e-5+beta_dot.*t3.*t21.*x.*y_dot.*3.84417e-5-beta_dot.*t3.*t21.*x_dot.*y.*8.94519e-5+beta_dot.*t15.*t19.*x.*y_dot.*3.84417e-5;
et80 = beta_dot.*t15.*t19.*x_dot.*y.*3.82338681e-2+gamma_dot.*t3.*t5.*t8.*y_dot.*1.323e-3-gamma_dot.*t5.*t8.*t15.*y_dot.*7.623e-3-gamma_dot.*t5.*t10.*t15.*y_dot.*1.26e-2-gamma_dot.*t3.*t8.*t20.*y_dot.*7.623e-3-gamma_dot.*t3.*t10.*t20.*y_dot.*1.26e-2-gamma_dot.*t11.*t14.*t19.*y_dot.*(6.3e+1./5.0e+2)-gamma_dot.*t14.*t19.*x.*x_dot.*1.60083e-5-beta_dot.*t20.*x.*y.*y_dot.*1.89e-4+beta_dot.*t22.*x.*y.*y_dot.*1.089e-3-gamma_dot.*t8.*t21.*y.*y_dot.*(6.3e+1./5.0e+2);
et81 = gamma_dot.*t14.*t19.*y.*y_dot.*(-3.83427681e-2)-t5.*t7.*t8.*t10.*t15.*(6.3e+1./1.0e+3)+t5.*t6.*t8.*t10.*t17.*(6.3e+1./1.0e+3)-t3.*t7.*t8.*t10.*t20.*(6.3e+1./1.0e+3)+t3.*t6.*t8.*t10.*t22.*(6.3e+1./1.0e+3)+t6.*t8.*t10.*t15.*t20.*(6.3e+1./5.0e+2)+t4.*t5.*t10.*t15.*x.*6.1803e-1+t3.*t4.*t10.*t20.*x.*6.1803e-1+t2.*t3.*t8.*t19.*y.*1.545075-t2.*t3.*t8.*t21.*y.*1.545075-t2.*t8.*t15.*t19.*y.*1.545075;
et82 = t6.*t8.*t14.*t19.*y.*(-2.412e-3)+t6.*t8.*t14.*t21.*y.*3.8115e-3+t6.*t8.*t16.*t19.*y.*7.623e-3+t4.*t14.*t19.*x.*y.*1.23155721-beta_dot.*gamma_dot.*t5.*t14.*x.*y.*1.89e-5+beta_dot.*gamma_dot.*t5.*t16.*x.*y.*3.845557095e-2+beta_dot.*gamma_dot.*t14.*t20.*x.*y.*3.833523645e-2+beta_dot.*t3.*t8.*t21.*x_dot.*y.*(6.3e+1./1.0e+3)-beta_dot.*t3.*t10.*t21.*x.*y_dot.*(6.3e+1./1.0e+3)+beta_dot.*t8.*t15.*t19.*x_dot.*y.*(6.3e+1./1.0e+3);
et83 = beta_dot.*t10.*t15.*t19.*x.*y_dot.*(-6.3e+1./1.0e+3)-beta_dot.*t5.*t16.*x.*y.*y_dot.*2.2239e-3-beta_dot.*t14.*t20.*x.*y.*y_dot.*1.1349e-3-gamma_dot.*t8.*t14.*t19.*y.*y_dot.*(6.3e+1./5.0e+2)+gamma_dot.*t5.*t15.*x.*x_dot.*y.*9.261e-4+gamma_dot.*t3.*t20.*x.*x_dot.*y.*9.261e-4-beta_dot.*gamma_dot.*t3.*t10.*t19.*x.*3.78e-4-beta_dot.*gamma_dot.*t5.*t11.*t16.*x.*(6.3e+1./5.0e+2)+beta_dot.*gamma_dot.*t3.*t10.*t21.*x.*9.1395e-3+beta_dot.*gamma_dot.*t10.*t15.*t19.*x.*2.8395e-3-beta_dot.*gamma_dot.*t11.*t14.*t20.*x.*(6.3e+1./5.0e+2);
out1 = [x_dot;t51.*(et1+et2+et3+et4+et5+et6+et7+et8+et9+et10+et11+et12+et13+et14+et15+et16+et17+et18+et19+et20+et21+et22+et23+et24+et25+et26);beta_dot;-t51.*(et27+et28+et29+et30+et31+et32+et33+et34+et35+et36+et37+et38);y_dot;t51.*(et39+et40+et41+et42+et43+et44+et45+et46+et47+et48+et49+et50+et51+et52+et53+et54+et55+et56+et57+et58+et59+et60+et61+et62+et63+et64+et65);gamma_dot;t51.*(et66+et67+et68+et69+et70+et71+et72+et73+et74+et75+et76+et77+et78+et79+et80+et81+et82+et83)];

== matlab function Linear_Moving_Setpoint_SS_PID/x_Setpoint_Function ==
  data: t input; x_setpoint_symfun output
function x_setpoint_symfun = x_setpoint(t)
%#codegen

%    This function was generated by the Symbolic Math Toolbox version 9.0.
%    08-Nov-2021 16:28:31

t2 = t.*pi.*2.0;
x_setpoint_symfun = [sin(t2)./1.0e+1;(pi.*cos(t2))./5.0];

== matlab function Linear_Moving_Setpoint_SS_PID/y_Setpoint_Function ==
  data: t input; y_setpoint_symfun output
function y_setpoint_symfun = y_setpoint(t)
%#codegen

%    This function was generated by the Symbolic Math Toolbox version 9.0.
%    08-Nov-2021 16:28:31

t2 = t.*pi.*2.0;
t3 = pi./2.0;
t4 = t2+t3;
y_setpoint_symfun = [sin(t4)./1.0e+1;(pi.*cos(t4))./5.0];
